simulink model "model_bicycleRider"  (R2020a)
settings: Solver=VariableStepAuto  StartTime=0.0  StopTime=300  FixedStep=0.5  RelTol=1e-3
undefined symbols (not defined in the file): lTan, magnitude, rTan, slope_in, targetPower
libraries: simulink x1
settings Model: Creator=rosswilkinson  LastModifiedBy=rosswilkinson
settings DataIOCC: ExternalInput=[a.time, a.signals.values]  SignalLogging=off  InspectSignalLogs=on

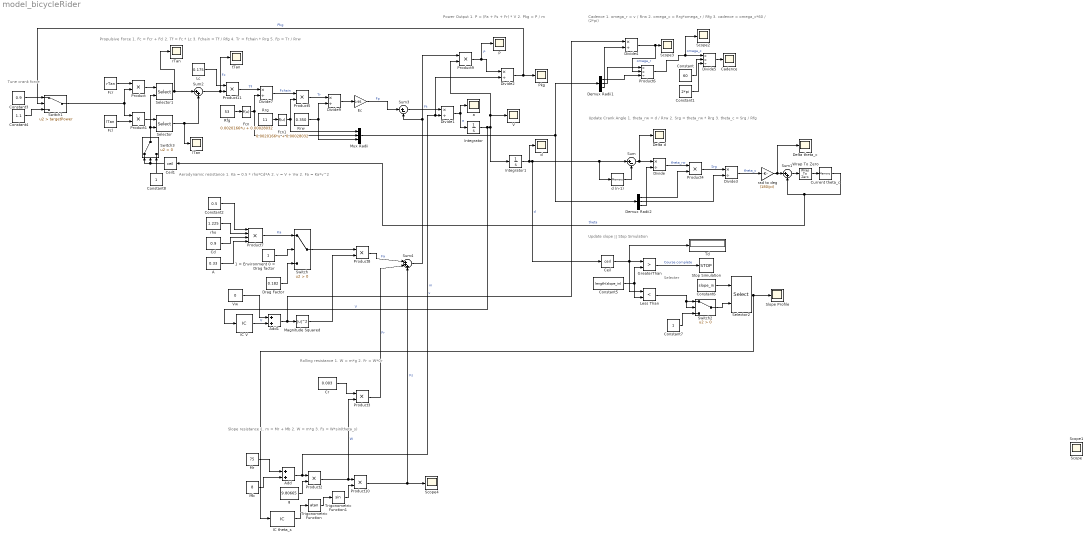
== system model_bicycleRider ==
  note: Tune crank force
  note: Selecter
  note: Rolling resistance
      | 1. W = m*g
      | 2. Fr = W*Cr
  note: Propulsive Force
      | 1. Fc = Fcr + Fcl
      | 2. Tf = Fc * Lc
      | 3. Fchain = Tf / Rfg
      | 4. Tr = Fchain * Rrg
      | 5. Fp = Tr / Rrw
  note: Update slope || Stop Simulation
  note: Slope resistance
      | 1. m = Mr + Mb
      | 2. W = m*g
      | 3. Fs = W*sin(theta_s)
  note: Power Output
      | 1. P = (Fa + Fs + Fr) * V
      | 2. Pkg = P / m
  note: Update Crank Angle
      | 1. theta_rw = d / Rrw
      | 2. Srg = theta_rw * Rrg
      | 3. theta_c = Srg / Rfg
  note: Aerodynamic resistance
      | 1. Ka = 0.5 * rho*Cd*A
      | 2. v = V + Vw
      | 2. Fa = Ka*v^2
  note: Cadence
      | 1. omega_r = v / Rrw
      | 2. omega_c = Rrg*omega_r / Rfg
      | 3. cadence = omega_c*60 / (2*pi)
  1 = Environment 0 = Drag factor : Constant
  A : Constant  Value=0.33
  Add : Sum
  Add1 : Sum
  Cadence : Scope
  Cd : Constant  Value=0.9
  Ceil : Rounding  Operator=ceil
  Ceil1 : Rounding  Operator=ceil
  Constant : Constant  Value=60
  Constant1 : Constant  Value=2*pi
  Constant2 : Constant  Value=0.5
  Constant3 : Constant  Value=0.9
  Constant4 : Constant  Value=1.1  SampleTime=Inf
  Constant5 : Constant  Value=length(slope_in)
  Constant6 : Constant  Value=slope_in
  Constant7 : Constant
  Constant8 : Constant
  Cr : Constant  Value=0.003
  Current theta_c : Memory
  Delta theta_c : Scope
  Delta d : Scope
  Demux Radii1 : Demux  Outputs=3
  Demux Radii2 : Demux  Outputs=3
  Divide{,1..4,7,9} (7 alike) : Product  Inputs=*/
  Divide5 : Product  Inputs=**/
  Drag Factor : Constant  Value=0.182
  Ec : Gain  Gain=0.95
  Fcl : Constant  Value=lTan
  Fcn : Fcn  Expr=0.0020166*u + 0.00028032
  Fcn1 : Fcn  Expr=0.0020166*u + 0.00028032
  Fcr : Constant  Value=rTan
  GreaterThan : RelationalOperator  Operator=>  OutDataTypeStr=boolean  RndMeth=Simplest
  IC V : InitialCondition  Value=0.1
  IC theta_s : InitialCondition  Value=slope_in(1)
  Integrator : Integrator
  Integrator1 : Integrator
  Lc : Constant  Value=0.175
  Less Than : RelationalOperator  Operator=<  OutDataTypeStr=boolean  RndMeth=Simplest
  Magnitude Squared : Math  Operator=magnitude^2  SaturateOnIntegerOverflow=on
  "Mb " : Constant  Value=8
  "Mr " : Constant  Value=75
  Mux Radii : Mux  Inputs=3
  P : Scope
  Pkg : Scope
  Product{,1..5,8..11} (10 alike) : Product
  Product6 : Product  Inputs=**/
  Product7 : Product  Inputs=4
  Rfg : Constant  Value=53
  Rrg : Constant  Value=11
  Rrw : Constant  Value=0.350
  Scope{,1..4} (5 alike) : Scope
  Selector : Selector  InputPortWidth=361  IndexOptions=Index vector (port)  Indices=[1 3]  OutputSizes=1
  Selector1 : Selector  InputPortWidth=361  IndexOptions=Index vector (port)  Indices=[1 3]  OutputSizes=1
  Selector2 : Selector  InputPortWidth=length(slope_in)  IndexOptions=Index vector (port)  Indices=[1 3]  OutputSizes=1
  Slope Profile : Scope
  Stop Simulation : Stop
  Sum : Sum  Inputs=|+-
  Sum1 : Sum  Inputs=|++
  Sum2 : Sum  Inputs=|++
  Sum3 : Sum  Inputs=|+-
  Sum4 : Sum  Inputs=|+++
  Switch : Switch  Criteria=u2 > Threshold
  Switch1 : Switch  Criteria=u2 > Threshold  Threshold=targetPower  OutDataTypeStr=double
  Switch2 : Switch  Criteria=u2 > Threshold
  Switch3 : Switch  Criteria=u2 > Threshold
  Td : Display
  Trigonometric Function : Trigonometry  Operator=atan
  Trigonometric Function1 : Trigonometry
  V : Scope
  Vw : Constant  Value=0
  Wrap To Zero : simulink/Discontinuities/Wrap To Zero  Threshold=2*pi
      settings: SourceProductBaseCode=SL
  a : Scope
  d : Scope
  d (n-1) : Memory
  g : Constant  Value=9.80665
  lTan : Scope
  rTan : Scope
  rad to deg : Gain  Gain=(180/pi)
  rho : Constant  Value=1.225
  tTan : Scope
  wires:
  "Mr "/1 -> Add/1
  Divide2/1 -> Pkg/1, Switch1/2  "Pkg"
  Sum3/1 -> Divide1/1  "Ft"
  Divide1/1 -> a/1, Integrator/1  "a"
  Rrw/1 -> Mux Radii/3, Divide9/2
  "Mb "/1 -> Add/2
  GreaterThan/1 -> Stop Simulation/1  "Course complete"
  Selector2/1 -> IC theta_s/1, Slope Profile/1
  Selector1/1 -> rTan/1, Sum2/1
  Sum/1 -> Divide/1, Delta d/1
  Selector/1 -> lTan/1, Sum2/2
  IC theta_s/1 -> Trigonometric Function/1
  Constant4/1 -> Switch1/3
  Constant3/1 -> Switch1/1
  Product9/1 -> P/1, Divide2/1  "P"
  Divide5/1 -> Cadence/1
  Lc/1 -> Product11/1
  Constant1/1 -> Divide5/3
  Constant/1 -> Divide5/2
  Product6/1 -> Scope2/1, Divide5/1  "omega_c"
  Divide4/1 -> Scope3/1, Product6/2  "omega_r"
  1 = Environment 0 = Drag factor/1 -> Switch/2
  Add1/1 -> Divide4/1, Magnitude Squared/1  "v"
  Product7/1 -> Switch/1  "Ka"
  Constant2/1 -> Product7/1
  Sum1/1 -> Wrap To Zero/1
  rad to deg/1 -> Delta theta_c/1, Sum1/1
  d (n-1)/1 -> Sum/2
  Wrap To Zero/1 -> Current theta_c/1
  Current theta_c/1 -> Ceil1/1, Sum1/2  "theta"
  Trigonometric Function/1 -> Trigonometric Function1/1
  Ceil/1 -> Td/1, GreaterThan/1, Less Than/1
  Constant5/1 -> GreaterThan/2, Less Than/2
  Product11/1 -> Divide7/1  "Tf"
  Divide7/1 -> Product5/1  "Fchain"
  Rrg/1 -> Fcn1/1
  Product5/1 -> Divide9/1  "Tr"
  rho/1 -> Product7/2
  Cd/1 -> Product7/3
  A/1 -> Product7/4
  Drag Factor/1 -> Switch/3
  Vw/1 -> Add1/1
  IC V/1 -> Add1/2  "V"
  Switch/1 -> Product8/1
  Magnitude Squared/1 -> Product8/2
  Cr/1 -> Product3/1
  Product3/1 -> Sum4/2  "Fr"
  Constant7/1 -> Switch2/3
  Switch2/1 -> Selector2/2
  Less Than/1 -> Switch2/2, Switch2/1
  Constant6/1 -> Selector2/1
  Add/1 -> Divide2/2, Divide1/2, Product2/1  "m"
  g/1 -> Product2/2
  Product2/1 -> Product3/2, Product10/1  "W"
  Product10/1 -> Scope4/1, Sum4/3  "Fs"
  Trigonometric Function1/1 -> Product10/2
  Sum2/1 -> tTan/1, Product11/2  "Fc"
  Ec/1 -> Sum3/1  "Fp"
  Divide9/1 -> Ec/1
  Product/1 -> Selector1/1
  Fcr/1 -> Product/1
  Fcl/1 -> Product1/2
  Product1/1 -> Selector/1
  Integrator1/1 -> d/1, d (n-1)/1, Sum/1, Ceil/1  "d"
  Sum4/1 -> Sum3/2, Product9/1
  Product8/1 -> Sum4/1  "Fa"
  Integrator/1 -> V/1, Product9/2, Integrator1/1, IC V/1  "V"
  Mux Radii/1 -> Demux Radii2/1, Demux Radii1/1
  Demux Radii1/1 -> Product6/3
  Demux Radii1/2 -> Product6/1
  Demux Radii1/3 -> Divide4/2
  Divide/1 -> Product4/1  "theta_rw"
  Demux Radii2/3 -> Divide/2
  Product4/1 -> Divide3/1  "Srg"
  Demux Radii2/1 -> Product4/2
  Demux Radii2/2 -> Divide3/2
  Divide3/1 -> rad to deg/1  "theta_c"
  Switch3/1 -> Selector1/2, Selector/2
  Constant8/1 -> Switch3/3
  Switch1/1 -> Product/2, Product1/1
  Rfg/1 -> Fcn/1
  Fcn/1 -> Divide7/2, Mux Radii/2
  Fcn1/1 -> Product5/2, Mux Radii/1
  Ceil1/1 -> Switch3/2, Switch3/1
